simulink model "lung_model_RLS_2018a"  (R2018a)
settings: Solver=VariableStepAuto  StartTime=0.0  StopTime=500  RelTol=1e-6  AbsTol=1e-3
values from neighbouring files (symbols this model uses):
  C = 0.02    [init_lung.m]
  C0 = 0.01    [init_lung.m]
  Delta = 0.01    [init_lung.m]
  p0 = (V0-C*PEEP)/(-C)    (= -95)    [init_lung.m]
  PEEP = 5    [init_lung.m]
  Pinsp = 20    [init_lung.m]
  R = 50    [init_lung.m]
  R0 = 10    [init_lung.m]
  Te = 2    [init_lung.m]
  Ti = 2    [init_lung.m]
  tt = 0:0.01:Ti    [init_lung.m]
  V0 = 2    [init_lung.m]
  yy = sin(2*pi/(Ti)*tt+pi*3/2)+1    [init_lung.m]
undefined symbols (not defined in the file or in its folder): DiscIntNeverNeededParam, rbf_data
libraries: simulink x2
settings Model: Creator=schauer  LastModifiedBy=schauer
settings SolverCC: ShapePreserveControl=EnableAll
settings DataIOCC: ReturnWorkspaceOutputs=on
settings SFSimCC: SimUseLocalCustomCode=on
settings RTWCC: RTWUseLocalCustomCode=on

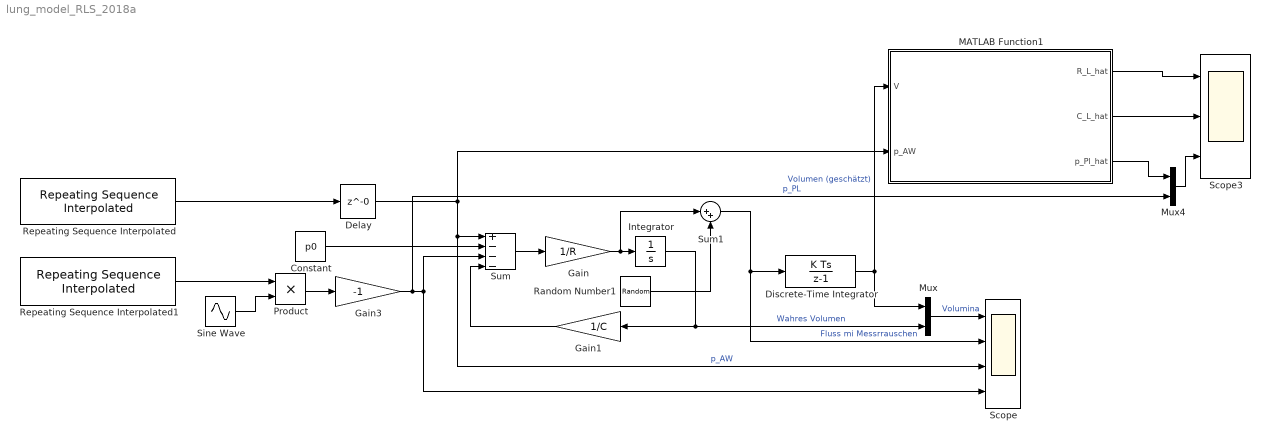
== system lung_model_RLS_2018a ==
  Constant : Constant  Value=p0
  Delay : Delay  DelayLength=0  InitialCondition=PEEP
  Discrete-Time Integrator : DiscreteIntegrator  gainval=1  SampleTime=Delta  ICPrevOutput=DiscIntNeverNeededParam  ICPrevScaledInput=DiscIntNeverNeededParam
  Gain : Gain  Gain=1/R
  Gain1 : Gain  Gain=1/C
  Gain3 : Gain  Gain=-1
  Integrator : Integrator  InitialCondition=V0
  MATLAB Function1 : MATLAB Function  TreatAsAtomicUnit=on  SystemSampleTime=Delta
  Mux : Mux  Inputs=2
  Mux4 : Mux  Inputs=2
  Product : Product
  Random Number1 : RandomNumber  Variance=0.0001  SampleTime=Delta
  Repeating Sequence Interpolated : simulink/Sources/Repeating Sequence Interpolated  OutValues=[PEEP Pinsp Pinsp PEEP PEEP]'  TimeValues=[0 Ti/8 Ti Ti+0.01 Ti+Te-Delta]'  LookUpMeth=Interpolation-Use End Values  tsamp=Delta  OutMin=[]  OutMax=[]  OutDataTypeStr=double  OutputDataTypeScalingMode=double  OutDataType=fixdt(0,8)  OutScaling=2^-10
  Repeating Sequence Interpolated1 : simulink/Sources/Repeating Sequence Interpolated  OutValues=[yy 0]*5  TimeValues=[tt Ti+Te-Delta]  LookUpMeth=Interpolation-Use End Values  tsamp=Delta  OutMin=[]  OutMax=[]  OutDataTypeStr=double  OutputDataTypeScalingMode=double  OutDataType=fixdt(0,8)  OutScaling=2^-10
  Scope : Scope  NumInputPorts=4
  Scope3 : Scope  NumInputPorts=3
  Sine Wave : Sin  Amplitude=0.5  Bias=0.5  Frequency=0.1*2*pi  SampleTime=0
  Sum : Sum  Inputs=+---
  Sum1 : Sum  Inputs=|++
  wires:
  MATLAB Function1/2(C_L_hat) -> Scope3/2
  MATLAB Function1/1(R_L_hat) -> Scope3/1
  Mux4/1 -> Scope3/3
  Sum/1 -> Gain/1
  Constant/1 -> Sum/2
  Gain1/1 -> Sum/4
  Delay/1 -> MATLAB Function1/2(p_AW), Scope/3, Sum/1  "p_AW"
  Integrator/1 -> Mux/2, Gain1/1  "Wahres Volumen"
  Repeating Sequence Interpolated/1 -> Delay/1
  Sine Wave/1 -> Product/2
  Random Number1/1 -> Sum1/2
  Mux/1 -> Scope/1  "Volumina"
  Repeating Sequence Interpolated1/1 -> Product/1
  Gain3/1 -> Mux4/2, Scope/4, Sum/3  "p_PL"
  Gain/1 -> Sum1/1, Integrator/1
  Product/1 -> Gain3/1
  Sum1/1 -> Scope/2, Discrete-Time Integrator/1  "Fluss mi Messrrauschen"
  Discrete-Time Integrator/1 -> Mux/1, MATLAB Function1/1(V)  "Volumen (geschätzt)"
  MATLAB Function1/3(p_Pl_hat) -> Mux4/1

== matlab function lung_model_RLS_2018a/MATLAB Function1 ==
  settings: updateMethod=DISCRETE
  data: V input; R_L_hat output; p_AW input; C_L_hat output; p_Pl_hat output; PEEP parameter; Ti parameter; Te parameter; Delta parameter; R0 parameter; C0 parameter; rbf_data parameter
function [R_L_hat,C_L_hat,p_Pl_hat] = rls_individual_lambda(V,p_AW,PEEP,Ti, Te, Delta,R0, C0,rbf_data)
%RBF parameter
o=rbf_data.o;%sigma
m=rbf_data.m;%mu's
n=rbf_data.n;%number of basis functions 

%Lambda settings
lambda_rc=0.999;
lambda_p_pl=0.98;
%Lambdas are 1 for R and C related parameters
Lambda=diag(sqrt([lambda_rc lambda_rc lambda_p_pl*ones(1,n)]));

%Numbers of samples used for initial LS
K=200;

%things to remember and initialisation 
persistent P_km1 Theta_hat_km1 p_AW_km1 V_km1 k i PHI Y

if isempty(P_km1)
    V_km1=0; 
    p_AW_km1=PEEP;
    k=0;%sample index
    i=1;%counter for initial LS, runs until K
    %determine inertial Theta_hat_km1 for R0 and C0
    alpha=-1/(R0*C0);
    beta=1/R0;
    a=exp(alpha*Delta);
    b=(beta/alpha)*(a-1);   
    Y=zeros(K,1);%measurement vector for initial LS
    PHI=zeros(K,n+2); %PHI matrix for initial LS / not used for RLS
    Theta_hat_km1 =[a b 0*randn(1,n)]';%output until LS finished
    %Dummy initial P0 Matrix, not really used
    P0=1;P_km1 = P0*diag([1 1 ones(1,n)].^2); 
end

l=floor((Delta*k)/(Ti+Te));
w=exp(-1/2*(((k*Delta-l*(Te+Ti))*ones(n,1)-m)/o).^2);
w=w+exp(-1/2*(((k*Delta-l*(Te+Ti))*ones(n,1)-(m+(Ti+Te)))/o).^2);

phi_k=[V_km1 
       (p_AW_km1-PEEP)
       -w];
y_k=V;

if i>K %normal RLS after LS has finished and determined the P0,Theta_hat_0
    L = (P_km1*phi_k)/(1+phi_k'*P_km1*phi_k);
    Theta_hat_k = Theta_hat_km1 + L*(y_k-phi_k'*Theta_hat_km1);
    P_k=Lambda^(-1)*(P_km1-L*phi_k'*P_km1)*Lambda^(-1);
elseif i<=K %Collect data fot the first K samples
    PHI(i,:)=phi_k';
    Y(i,:)=y_k;
    Theta_hat_k=Theta_hat_km1;
    P_k=P_km1;
else
    Theta_hat_k=Theta_hat_km1;
    P_k=P_km1;
end

%Solve LS if K samples have arrived
if i==K
    Theta_hat_k=PHI\Y;
    P_k=inv(PHI'*PHI);
end

%Solve for R_L and C_L
a=Theta_hat_k(1);b=Theta_hat_k(2);
RC=-1/(log(a)/Delta);
alpha=log(a)/Delta;
beta=b*alpha/(a-1);
R_L_hat=1/beta;
C_L_hat=RC/R_L_hat;
%Estimation of p_Pl
p_Pl_hat = Theta_hat_k(3:end)'*w/Theta_hat_k(2);

%Updates
Theta_hat_km1=Theta_hat_k;
P_km1=P_k;
p_AW_km1=p_AW;
V_km1=V;
k=k+1;
i=i+1;
end
